simulink model "GradingSys"  (R2020a)
settings: Solver=FixedStepDiscrete  StartTime=0.0  StopTime=10.0  RelTol=1e-3
settings Model: Creator=yomna  LastModifiedBy=yomna
settings OptimizationCC: DefaultParameterBehavior=Inlined  EnhancedBackFolding=on  PassReuseOutputArgsAs=Individual arguments  ZeroExternalMemoryAtStartup=off  ZeroInternalMemoryAtStartup=off  OptimizeBlockOrder=speed  DifferentSizesBufferReuse=on  OptimizationCustomize=off  EfficientTunableParamExpr=on
settings DebuggingCC: UnderspecifiedInitializationDetection=Classic  MergeDetectMultiDrivingBlocksExec=none  ParameterTunabilityLossMsg=error
settings ModelReferenceCC: PropagateSignalLabelsOutOfModel=off
settings SFSimCC: MATLABDynamicMemAlloc=off
settings RTWCC: SystemTargetFile=ert.tlc  GenCodeOnly=on  TemplateMakefile=ert_default_tmf  GenerateReport=on  IncludeHyperlinkInReport=on  LaunchReport=on  GenerateTraceInfo=on  GenerateTraceReport=on  GenerateTraceReportSl=on  GenerateTraceReportSf=on  GenerateTraceReportEml=on
settings CodeAppCC: ForceParamTrailComments=on  IgnoreCustomStorageClasses=off  OperatorAnnotations=on  SimulinkDataObjDesc=on  SFDataObjDesc=on  InsertBlockDesc=on
settings ERTTargetCC: TargetLangStandard=C99 (ISO)  GenerateSampleERTMain=on  InlinedParameterPlacement=NonHierarchical  ERTCustomFileTemplate=example_file_process.tlc

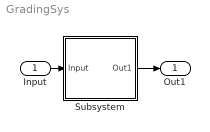
== system GradingSys ==
  Input : Inport
  Subsystem : Subsystem
  Out1 : Outport
  wires:
  Subsystem/1(Out1) -> Out1/1
  Input/1 -> Subsystem/1(Input)

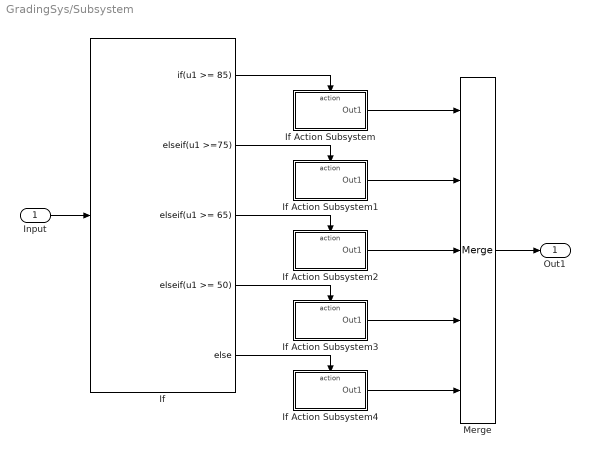
== system GradingSys/Subsystem ==
  Input : Inport  OutDataTypeStr=double
  If : If  IfExpression=u1 >= 85  ElseIfExpressions=u1 >=75 , u1 >= 65 , u1 >= 50
  If Action Subsystem : Subsystem  TreatAsAtomicUnit=on
  If Action Subsystem1 : Subsystem  TreatAsAtomicUnit=on
  If Action Subsystem2 : Subsystem  TreatAsAtomicUnit=on
  If Action Subsystem3 : Subsystem  TreatAsAtomicUnit=on
  If Action Subsystem4 : Subsystem  TreatAsAtomicUnit=on
  Merge : Merge  Inputs=5
  Out1 : Outport
  wires:
  If/5 -> If Action Subsystem4/Action
  Input/1 -> If/1
  If/1 -> If Action Subsystem/Action
  If/3 -> If Action Subsystem2/Action
  If/2 -> If Action Subsystem1/Action
  If Action Subsystem2/1(Out1) -> Merge/3
  Merge/1 -> Out1/1
  If Action Subsystem/1(Out1) -> Merge/1
  If Action Subsystem4/1(Out1) -> Merge/5
  If Action Subsystem3/1(Out1) -> Merge/4
  If Action Subsystem1/1(Out1) -> Merge/2
  If/4 -> If Action Subsystem3/Action

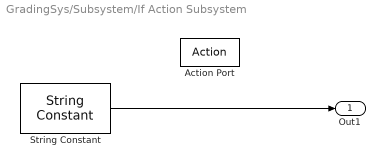
== system GradingSys/Subsystem/If Action Subsystem ==
  Action Port : ActionPort  ActionPortLabel=if(u1 >= 85)
  String Constant : StringConstant  String="\"Distinct!\""
  Out1 : Outport
  wires:
  String Constant/1 -> Out1/1

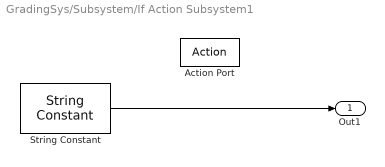
== system GradingSys/Subsystem/If Action Subsystem1 ==
  Action Port : ActionPort  ActionPortLabel=elseif(u1 >=75 )
  String Constant : StringConstant  String="\"Very Good\""
  Out1 : Outport
  wires:
  String Constant/1 -> Out1/1

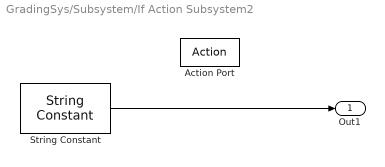
== system GradingSys/Subsystem/If Action Subsystem2 ==
  Action Port : ActionPort  ActionPortLabel=elseif( u1 >= 65 )
  String Constant : StringConstant  String="\"Good\""
  Out1 : Outport
  wires:
  String Constant/1 -> Out1/1

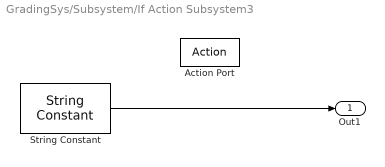
== system GradingSys/Subsystem/If Action Subsystem3 ==
  Action Port : ActionPort  ActionPortLabel=elseif( u1 >= 50)
  String Constant : StringConstant  String="\"Pass\""
  Out1 : Outport
  wires:
  String Constant/1 -> Out1/1

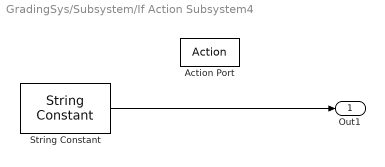
== system GradingSys/Subsystem/If Action Subsystem4 ==
  Action Port : ActionPort  ActionPortLabel=else
  String Constant : StringConstant  String="\"Fail\""
  Out1 : Outport
  wires:
  String Constant/1 -> Out1/1
